simulink model "lab6_1"  (R2020b)
settings: Solver=VariableStepAuto  StartTime=0.0  StopTime=350000  MaxStep=0.01  RelTol=1e-3
InitFcn:
  | lambda = 5;
  | 
  | a0 = 1; a1 = 5;
  | b0 = 6; b1 = 1;
  | k1 = 0.6; k0 = 0.09;
  | 
  | A = [-a1 1; -a0 0];
  | b = [b1; b0];
  | 
  | A0 = [-k1 1; -k0 0];
  | 
  | theta = [k0-a0; k1-a1; b0; b1];
  | 
  | C = [1 0]
settings Model: SimulationMode=accelerator  Creator=Eeer12  LastModifiedBy=Eugene

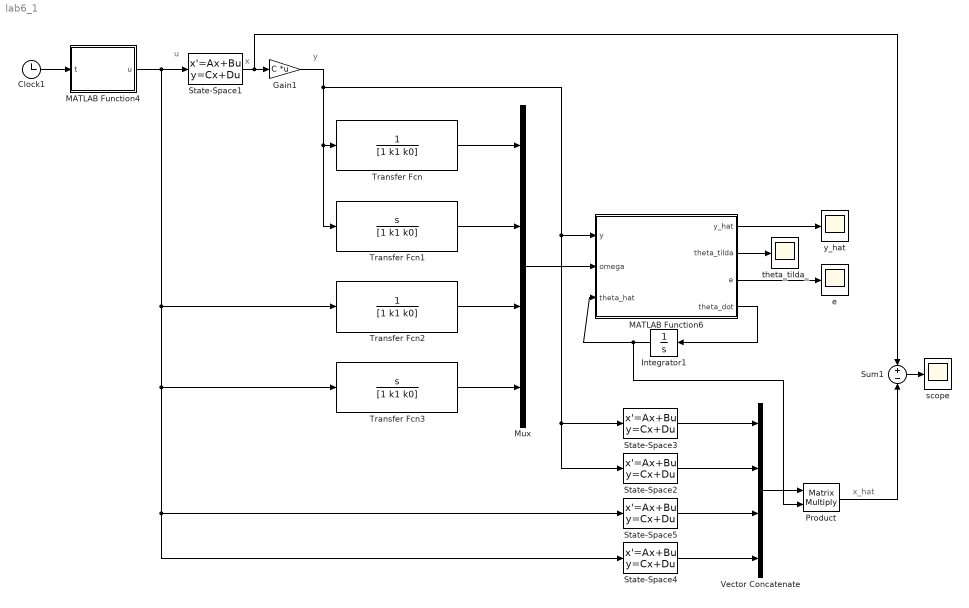
== system lab6_1 ==
  note: x_hat
  note: u
  note: y
  note: x
  Clock1 : Clock
  Gain1 : Gain  Gain=C  Multiplication=Matrix(K*u)
  Integrator1 : Integrator  InitialCondition=[0; 0; 0; 0]
  MATLAB Function4 : MATLAB Function  TreatAsAtomicUnit=on
  MATLAB Function6 : MATLAB Function  TreatAsAtomicUnit=on
  Mux : Mux
  Product : Product  Multiplication=Matrix(*)
  State-Space1 : StateSpace  A=A  B=b  C=eye(2)  D=[0; 0]  InitialCondition=[0; 0]
  State-Space2 : StateSpace  A=A0  B=[1; 0]  C=eye(2)  D=[0; 0]  InitialCondition=[0; 0]
  State-Space3 : StateSpace  A=A0  B=[0; 1]  C=eye(2)  D=[0; 0]  InitialCondition=[0; 0]
  State-Space4 : StateSpace  A=A0  B=[1; 0]  C=eye(2)  D=[0; 0]  InitialCondition=[0; 0]
  State-Space5 : StateSpace  A=A0  B=[0; 1]  C=eye(2)  D=[0; 0]  InitialCondition=[0; 0]
  Sum1 : Sum  Inputs=+-
  Transfer Fcn : TransferFcn  Denominator=[1 k1 k0]
  Transfer Fcn1 : TransferFcn  Numerator=[1 0]  Denominator=[1 k1 k0]
  Transfer Fcn2 : TransferFcn  Denominator=[1 k1 k0]
  Transfer Fcn3 : TransferFcn  Numerator=[1 0]  Denominator=[1 k1 k0]
  Vector Concatenate : Concatenate  NumInputs=4  Mode=Multidimensional array  ConcatenateDimension=2
  e : Scope
  scope : Scope
  theta_tilda_ : Scope
  y_hat : Scope
  wires:
  State-Space1/1 -> Sum1/1, Gain1/1
  Clock1/1 -> MATLAB Function4/1(t)
  MATLAB Function4/1(u) -> Transfer Fcn2/1, State-Space4/1, State-Space5/1, Transfer Fcn3/1, State-Space1/1
  Gain1/1 -> State-Space2/1, State-Space3/1, MATLAB Function6/1(y), Transfer Fcn1/1, Transfer Fcn/1
  Transfer Fcn/1 -> Mux/1
  Transfer Fcn1/1 -> Mux/2
  Transfer Fcn2/1 -> Mux/3
  Transfer Fcn3/1 -> Mux/4
  Mux/1 -> MATLAB Function6/2(omega)
  MATLAB Function6/4(theta_dot) -> Integrator1/1
  Integrator1/1 -> Product/2, MATLAB Function6/3(theta_hat)
  MATLAB Function6/1(y_hat) -> y_hat/1
  MATLAB Function6/2(theta_tilda) -> theta_tilda_/1
  MATLAB Function6/3(e) -> e/1
  State-Space4/1 -> Vector Concatenate/4
  State-Space5/1 -> Vector Concatenate/3
  State-Space2/1 -> Vector Concatenate/2
  State-Space3/1 -> Vector Concatenate/1
  Vector Concatenate/1 -> Product/1
  Product/1 -> Sum1/2
  Sum1/1 -> scope/1

== matlab function lab6_1/MATLAB Function4 ==
  data: t input; u output
function u = fcn(t)

u = sin(t)+0.5*cos(2*t);

== matlab function lab6_1/MATLAB Function6 ==
  data: y_hat output; theta_tilda output; e output; y input; omega input; theta_hat input; theta_dot output; theta parameter
function [y_hat, theta_tilda, e, theta_dot] = fcn(y, omega, theta_hat, theta)

theta_tilda = theta - theta_hat;

gamma = 10;

y_hat = theta_hat'*omega;

e = y - y_hat;

theta_dot = gamma*omega*e;
